simulink subsystem "joystick_subscriber"  (R2025b)
settings: Solver=VariableStepAuto  StartTime=0.0  StopTime=10.0  RelTol=1e-3
libraries: ros2lib x1
settings Model: Creator=vulcangrip  LastModifiedBy=vulcangrip

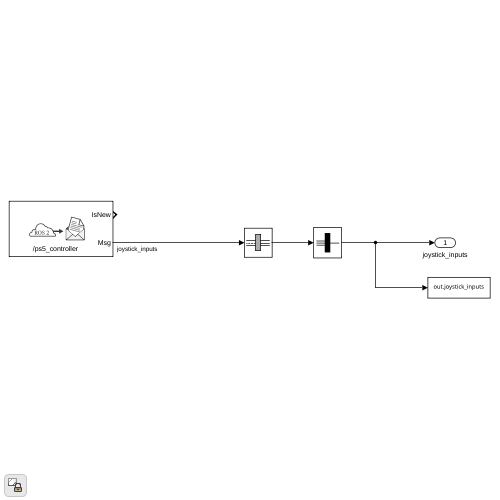
[thumbnail: Simulink's stored preview of the top-level diagram]
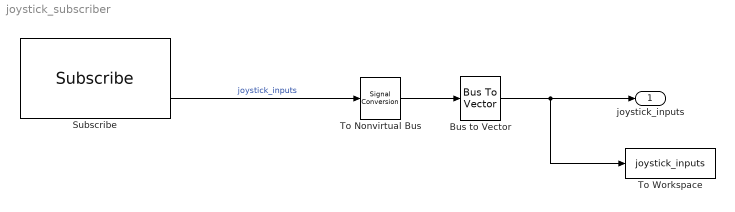
== system joystick_subscriber ==
  Bus to Vector : BusToVector
  Subscribe : ros2lib/Subscribe  topicSource=Specify your own  topic=/ps5_controller  messageType=remote_control_interface/Gamepad  sampleTime=1/60  QOSHistory=Keep last  QOSDepth=10  QOSReliability=Reliable  QOSDurability=Volatile  QOSDeadline=Inf  QOSLifespan=Inf  QOSLiveliness=Automatic  QOSLeaseDuration=Inf  QOSAvoidROSNamespaceConventions=off
  To Nonvirtual Bus : SignalConversion  ConversionOutput=Virtual bus  OverrideOpt=off
  To Workspace : ToWorkspace  VariableName=joystick_inputs  SaveFormat=Timeseries  SampleTime=-1
  joystick_inputs : Outport
  wires:
  Subscribe/2 -> To Nonvirtual Bus/1  "joystick_inputs"
  To Nonvirtual Bus/1 -> Bus to Vector/1
  Bus to Vector/1 -> joystick_inputs/1, To Workspace/1
